simulink model "dSAW"  (R2019a)
settings: Solver=FixedStepAuto  StartTime=0.0  StopTime=40  FixedStep=0.001  MaxStep=0.01  RelTol=1e-3  AbsTol=1e-3  EnableMultiTasking=on
values from neighbouring files (symbols this model uses):
  alp = data(:,1)    [Main.m]
  be_gap = 23    [Main.m]
  cd = data(:,3)    [Main.m]
  chord_lengths = [61.1183,64.3430,68.0127,71.9324,                 75.9071,79.7418,83.2415,86.2112,                 88.4559,89.7806,89.9903,88.8900]    [Main.m]
  cl = data(:,2)    [Main.m]
  epsilon = 0.2010    (= 0.201)    [Main.m]
  gamma_amp = 0.1188    [Main.m]
  gamma_o = -0.1345    [Main.m]
undefined symbols (not defined in the file or in its folder): X, Y, Z
libraries: sm_lib x168, nesl_utility x109, dspindex x2
(part 3 of 3)

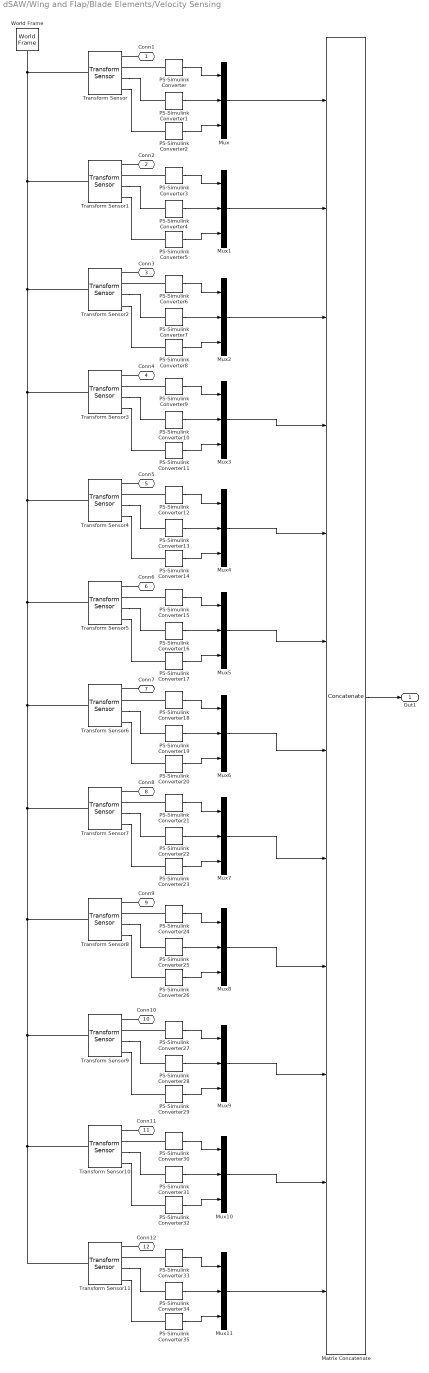
== system dSAW/Wing and Flap/Blade Elements/Velocity Sensing ==
  Matrix Concatenate : Concatenate  NumInputs=12  Mode=Multidimensional array  ConcatenateDimension=2
  Mux{,1..11} (12 alike) : Mux  Inputs=3
  PS-Simulink Converter{,1..35} (36 alike) : nesl_utility/PS-Simulink Converter  PhysicalDomain=network_engine_domain  SubClassName=ps_output  LeftPortType=input  RightPortType=output  PseudoPeriodic=off  Frequencies=[]  Unit=1  AffineConversion=off
  Transform Sensor{,1..11} (12 alike) : sm_lib/Frames and Transforms/Transform Sensor  MeasurementFrame=NonRotatingFollower  SenseAngle=off  SenseAxis=off  SenseAngle1=off  SenseAngle2=off  SenseAngle3=off  SenseQ=off  SenseR=off  SenseOmegaX=off  SenseOmegaY=off  SenseOmegaZ=off  SenseOmega1=off  SenseOmega2=off  SenseOmega3=off  SenseQDot=off  SenseRDot=off  SenseAlphaX=off  SenseAlphaY=off  SenseAlphaZ=off  SenseAlpha1=off  SenseAlpha2=off  SenseAlpha3=off  SenseQDDot=off  SenseRDDot=off  SenseX=off  SenseY=off  SenseZ=off  SenseRad=off  SenseAzim=off  SenseDist=off  SenseInc=off  SenseXDot=on  SenseYDot=on  SenseZDot=on  SenseRadDot=off  SenseAzimDot=off  SenseDistDot=off  SenseIncDot=off  SenseXDDot=off  SenseYDDot=off  SenseZDDot=off  SenseRadDDot=off  SenseAzimDDot=off  SenseDistDDot=off  SenseIncDDot=off
  World Frame : sm_lib/Frames and Transforms/World Frame
  Conn1 : PMIOPort  Side=Left
  Conn2 : PMIOPort  Port=2  Side=Left
  Conn3 : PMIOPort  Port=3  Side=Left
  Conn4 : PMIOPort  Port=4  Side=Left
  Conn5 : PMIOPort  Port=5  Side=Left
  Conn6 : PMIOPort  Port=6  Side=Left
  Conn7 : PMIOPort  Port=7  Side=Left
  Conn8 : PMIOPort  Port=8  Side=Left
  Conn9 : PMIOPort  Port=9  Side=Left
  Conn10 : PMIOPort  Port=10  Side=Left
  Conn11 : PMIOPort  Port=11  Side=Left
  Conn12 : PMIOPort  Port=12  Side=Left
  Out1 : Outport
  wires:
  PS-Simulink Converter1/1 -> Mux/2
  PS-Simulink Converter/1 -> Mux/1
  PS-Simulink Converter2/1 -> Mux/3
  Matrix Concatenate/1 -> Out1/1
  Mux/1 -> Matrix Concatenate/1
  Mux1/1 -> Matrix Concatenate/2
  PS-Simulink Converter3/1 -> Mux1/1
  PS-Simulink Converter4/1 -> Mux1/2
  PS-Simulink Converter5/1 -> Mux1/3
  PS-Simulink Converter6/1 -> Mux2/1
  PS-Simulink Converter7/1 -> Mux2/2
  PS-Simulink Converter8/1 -> Mux2/3
  PS-Simulink Converter9/1 -> Mux3/1
  PS-Simulink Converter10/1 -> Mux3/2
  PS-Simulink Converter11/1 -> Mux3/3
  PS-Simulink Converter12/1 -> Mux4/1
  PS-Simulink Converter13/1 -> Mux4/2
  PS-Simulink Converter14/1 -> Mux4/3
  PS-Simulink Converter15/1 -> Mux5/1
  PS-Simulink Converter16/1 -> Mux5/2
  PS-Simulink Converter17/1 -> Mux5/3
  PS-Simulink Converter18/1 -> Mux6/1
  PS-Simulink Converter19/1 -> Mux6/2
  PS-Simulink Converter20/1 -> Mux6/3
  PS-Simulink Converter21/1 -> Mux7/1
  PS-Simulink Converter22/1 -> Mux7/2
  PS-Simulink Converter23/1 -> Mux7/3
  Mux2/1 -> Matrix Concatenate/3
  Mux3/1 -> Matrix Concatenate/4
  Mux4/1 -> Matrix Concatenate/5
  Mux5/1 -> Matrix Concatenate/6
  Mux6/1 -> Matrix Concatenate/7
  Mux7/1 -> Matrix Concatenate/8
  PS-Simulink Converter26/1 -> Mux8/3
  PS-Simulink Converter25/1 -> Mux8/2
  PS-Simulink Converter24/1 -> Mux8/1
  PS-Simulink Converter27/1 -> Mux9/1
  PS-Simulink Converter28/1 -> Mux9/2
  PS-Simulink Converter29/1 -> Mux9/3
  PS-Simulink Converter32/1 -> Mux10/3
  PS-Simulink Converter31/1 -> Mux10/2
  PS-Simulink Converter30/1 -> Mux10/1
  Mux8/1 -> Matrix Concatenate/9
  Mux9/1 -> Matrix Concatenate/10
  Mux10/1 -> Matrix Concatenate/11
  Mux11/1 -> Matrix Concatenate/12
  PS-Simulink Converter33/1 -> Mux11/1
  PS-Simulink Converter34/1 -> Mux11/2
  PS-Simulink Converter35/1 -> Mux11/3
  connections:
  Transform Sensor/LConn1 -- Transform Sensor11/LConn1 -- Transform Sensor10/LConn1 -- Transform Sensor9/LConn1 -- Transform Sensor8/LConn1 -- Transform Sensor7/LConn1 -- Transform Sensor6/LConn1 -- Transform Sensor5/LConn1 -- Transform Sensor4/LConn1 -- Transform Sensor3/LConn1 -- Transform Sensor2/LConn1 -- Transform Sensor1/LConn1 -- World Frame/RConn1
  Conn1/RConn1 -- Transform Sensor/RConn1
  PS-Simulink Converter/LConn1 -- Transform Sensor/RConn2
  Transform Sensor/RConn3 -- PS-Simulink Converter1/LConn1
  Transform Sensor/RConn4 -- PS-Simulink Converter2/LConn1
  Transform Sensor1/RConn4 -- PS-Simulink Converter5/LConn1
  PS-Simulink Converter3/LConn1 -- Transform Sensor1/RConn2
  Transform Sensor1/RConn3 -- PS-Simulink Converter4/LConn1
  Conn2/RConn1 -- Transform Sensor1/RConn1
  PS-Simulink Converter6/LConn1 -- Transform Sensor2/RConn2
  Transform Sensor2/RConn4 -- PS-Simulink Converter8/LConn1
  Transform Sensor2/RConn3 -- PS-Simulink Converter7/LConn1
  PS-Simulink Converter9/LConn1 -- Transform Sensor3/RConn2
  Transform Sensor3/RConn4 -- PS-Simulink Converter11/LConn1
  Transform Sensor3/RConn3 -- PS-Simulink Converter10/LConn1
  PS-Simulink Converter12/LConn1 -- Transform Sensor4/RConn2
  Transform Sensor4/RConn4 -- PS-Simulink Converter14/LConn1
  Transform Sensor4/RConn3 -- PS-Simulink Converter13/LConn1
  PS-Simulink Converter15/LConn1 -- Transform Sensor5/RConn2
  Transform Sensor5/RConn4 -- PS-Simulink Converter17/LConn1
  Transform Sensor5/RConn3 -- PS-Simulink Converter16/LConn1
  PS-Simulink Converter18/LConn1 -- Transform Sensor6/RConn2
  Transform Sensor6/RConn4 -- PS-Simulink Converter20/LConn1
  Transform Sensor6/RConn3 -- PS-Simulink Converter19/LConn1
  PS-Simulink Converter21/LConn1 -- Transform Sensor7/RConn2
  Transform Sensor7/RConn4 -- PS-Simulink Converter23/LConn1
  Transform Sensor7/RConn3 -- PS-Simulink Converter22/LConn1
  Conn3/RConn1 -- Transform Sensor2/RConn1
  Conn4/RConn1 -- Transform Sensor3/RConn1
  Conn5/RConn1 -- Transform Sensor4/RConn1
  Conn6/RConn1 -- Transform Sensor5/RConn1
  Conn7/RConn1 -- Transform Sensor6/RConn1
  Conn8/RConn1 -- Transform Sensor7/RConn1
  Conn9/RConn1 -- Transform Sensor8/RConn1
  Transform Sensor8/RConn3 -- PS-Simulink Converter25/LConn1
  Transform Sensor8/RConn4 -- PS-Simulink Converter26/LConn1
  PS-Simulink Converter24/LConn1 -- Transform Sensor8/RConn2
  PS-Simulink Converter27/LConn1 -- Transform Sensor9/RConn2
  Transform Sensor9/RConn4 -- PS-Simulink Converter29/LConn1
  Transform Sensor9/RConn3 -- PS-Simulink Converter28/LConn1
  Conn10/RConn1 -- Transform Sensor9/RConn1
  Transform Sensor10/RConn3 -- PS-Simulink Converter31/LConn1
  Transform Sensor10/RConn4 -- PS-Simulink Converter32/LConn1
  Conn11/RConn1 -- Transform Sensor10/RConn1
  PS-Simulink Converter30/LConn1 -- Transform Sensor10/RConn2
  Conn12/RConn1 -- Transform Sensor11/RConn1
  PS-Simulink Converter33/LConn1 -- Transform Sensor11/RConn2
  Transform Sensor11/RConn4 -- PS-Simulink Converter35/LConn1
  Transform Sensor11/RConn3 -- PS-Simulink Converter34/LConn1

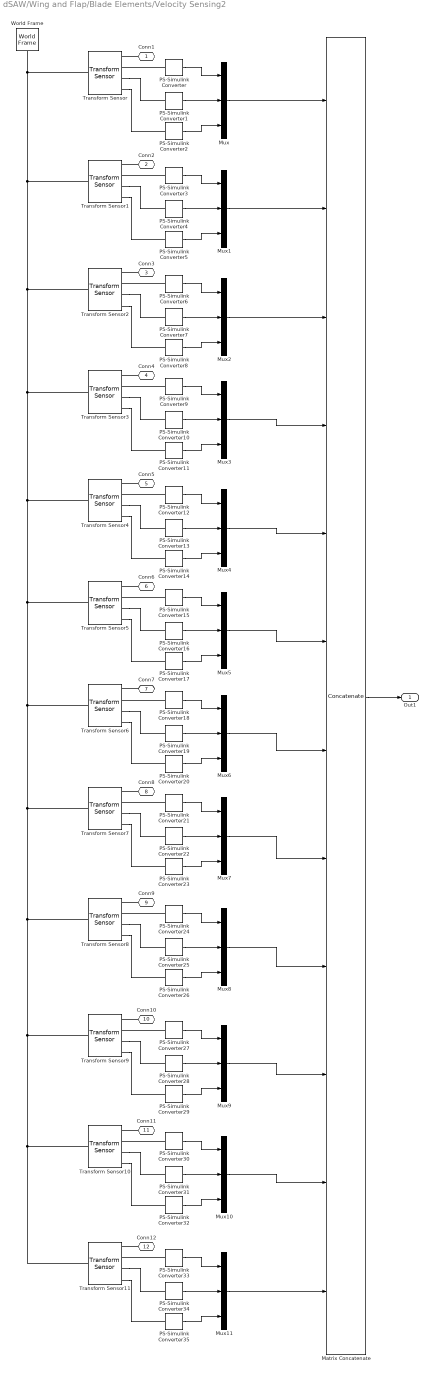
== system dSAW/Wing and Flap/Blade Elements/Velocity Sensing2 ==
  Matrix Concatenate : Concatenate  NumInputs=12  Mode=Multidimensional array  ConcatenateDimension=2
  Mux{,1..11} (12 alike) : Mux  Inputs=3
  PS-Simulink Converter{,1..35} (36 alike) : nesl_utility/PS-Simulink Converter  PhysicalDomain=network_engine_domain  SubClassName=ps_output  LeftPortType=input  RightPortType=output  PseudoPeriodic=off  Frequencies=[]  Unit=1  AffineConversion=off
  Transform Sensor{,1..11} (12 alike) : sm_lib/Frames and Transforms/Transform Sensor  MeasurementFrame=NonRotatingFollower  SenseAngle=off  SenseAxis=off  SenseAngle1=off  SenseAngle2=off  SenseAngle3=off  SenseQ=off  SenseR=off  SenseOmegaX=off  SenseOmegaY=off  SenseOmegaZ=off  SenseOmega1=off  SenseOmega2=off  SenseOmega3=off  SenseQDot=off  SenseRDot=off  SenseAlphaX=off  SenseAlphaY=off  SenseAlphaZ=off  SenseAlpha1=off  SenseAlpha2=off  SenseAlpha3=off  SenseQDDot=off  SenseRDDot=off  SenseX=off  SenseY=off  SenseZ=off  SenseRad=off  SenseAzim=off  SenseDist=off  SenseInc=off  SenseXDot=on  SenseYDot=on  SenseZDot=on  SenseRadDot=off  SenseAzimDot=off  SenseDistDot=off  SenseIncDot=off  SenseXDDot=off  SenseYDDot=off  SenseZDDot=off  SenseRadDDot=off  SenseAzimDDot=off  SenseDistDDot=off  SenseIncDDot=off
  World Frame : sm_lib/Frames and Transforms/World Frame
  Conn1 : PMIOPort  Side=Left
  Conn2 : PMIOPort  Port=2  Side=Left
  Conn3 : PMIOPort  Port=3  Side=Left
  Conn4 : PMIOPort  Port=4  Side=Left
  Conn5 : PMIOPort  Port=5  Side=Left
  Conn6 : PMIOPort  Port=6  Side=Left
  Conn7 : PMIOPort  Port=7  Side=Left
  Conn8 : PMIOPort  Port=8  Side=Left
  Conn9 : PMIOPort  Port=9  Side=Left
  Conn10 : PMIOPort  Port=10  Side=Left
  Conn11 : PMIOPort  Port=11  Side=Left
  Conn12 : PMIOPort  Port=12  Side=Left
  Out1 : Outport
  wires:
  PS-Simulink Converter1/1 -> Mux/2
  PS-Simulink Converter/1 -> Mux/1
  PS-Simulink Converter2/1 -> Mux/3
  Matrix Concatenate/1 -> Out1/1
  Mux/1 -> Matrix Concatenate/1
  Mux1/1 -> Matrix Concatenate/2
  PS-Simulink Converter3/1 -> Mux1/1
  PS-Simulink Converter4/1 -> Mux1/2
  PS-Simulink Converter5/1 -> Mux1/3
  PS-Simulink Converter6/1 -> Mux2/1
  PS-Simulink Converter7/1 -> Mux2/2
  PS-Simulink Converter8/1 -> Mux2/3
  PS-Simulink Converter9/1 -> Mux3/1
  PS-Simulink Converter10/1 -> Mux3/2
  PS-Simulink Converter11/1 -> Mux3/3
  PS-Simulink Converter12/1 -> Mux4/1
  PS-Simulink Converter13/1 -> Mux4/2
  PS-Simulink Converter14/1 -> Mux4/3
  PS-Simulink Converter15/1 -> Mux5/1
  PS-Simulink Converter16/1 -> Mux5/2
  PS-Simulink Converter17/1 -> Mux5/3
  PS-Simulink Converter18/1 -> Mux6/1
  PS-Simulink Converter19/1 -> Mux6/2
  PS-Simulink Converter20/1 -> Mux6/3
  PS-Simulink Converter21/1 -> Mux7/1
  PS-Simulink Converter22/1 -> Mux7/2
  PS-Simulink Converter23/1 -> Mux7/3
  Mux2/1 -> Matrix Concatenate/3
  Mux3/1 -> Matrix Concatenate/4
  Mux4/1 -> Matrix Concatenate/5
  Mux5/1 -> Matrix Concatenate/6
  Mux6/1 -> Matrix Concatenate/7
  Mux7/1 -> Matrix Concatenate/8
  PS-Simulink Converter26/1 -> Mux8/3
  PS-Simulink Converter25/1 -> Mux8/2
  PS-Simulink Converter24/1 -> Mux8/1
  PS-Simulink Converter27/1 -> Mux9/1
  PS-Simulink Converter28/1 -> Mux9/2
  PS-Simulink Converter29/1 -> Mux9/3
  PS-Simulink Converter32/1 -> Mux10/3
  PS-Simulink Converter31/1 -> Mux10/2
  PS-Simulink Converter30/1 -> Mux10/1
  Mux8/1 -> Matrix Concatenate/9
  Mux9/1 -> Matrix Concatenate/10
  Mux10/1 -> Matrix Concatenate/11
  Mux11/1 -> Matrix Concatenate/12
  PS-Simulink Converter33/1 -> Mux11/1
  PS-Simulink Converter34/1 -> Mux11/2
  PS-Simulink Converter35/1 -> Mux11/3
  connections:
  Transform Sensor/LConn1 -- Transform Sensor11/LConn1 -- Transform Sensor10/LConn1 -- Transform Sensor9/LConn1 -- Transform Sensor8/LConn1 -- Transform Sensor7/LConn1 -- Transform Sensor6/LConn1 -- Transform Sensor5/LConn1 -- Transform Sensor4/LConn1 -- Transform Sensor3/LConn1 -- Transform Sensor2/LConn1 -- Transform Sensor1/LConn1 -- World Frame/RConn1
  Conn1/RConn1 -- Transform Sensor/RConn1
  PS-Simulink Converter/LConn1 -- Transform Sensor/RConn2
  Transform Sensor/RConn3 -- PS-Simulink Converter1/LConn1
  Transform Sensor/RConn4 -- PS-Simulink Converter2/LConn1
  Transform Sensor1/RConn4 -- PS-Simulink Converter5/LConn1
  PS-Simulink Converter3/LConn1 -- Transform Sensor1/RConn2
  Transform Sensor1/RConn3 -- PS-Simulink Converter4/LConn1
  Conn2/RConn1 -- Transform Sensor1/RConn1
  PS-Simulink Converter6/LConn1 -- Transform Sensor2/RConn2
  Transform Sensor2/RConn4 -- PS-Simulink Converter8/LConn1
  Transform Sensor2/RConn3 -- PS-Simulink Converter7/LConn1
  PS-Simulink Converter9/LConn1 -- Transform Sensor3/RConn2
  Transform Sensor3/RConn4 -- PS-Simulink Converter11/LConn1
  Transform Sensor3/RConn3 -- PS-Simulink Converter10/LConn1
  PS-Simulink Converter12/LConn1 -- Transform Sensor4/RConn2
  Transform Sensor4/RConn4 -- PS-Simulink Converter14/LConn1
  Transform Sensor4/RConn3 -- PS-Simulink Converter13/LConn1
  PS-Simulink Converter15/LConn1 -- Transform Sensor5/RConn2
  Transform Sensor5/RConn4 -- PS-Simulink Converter17/LConn1
  Transform Sensor5/RConn3 -- PS-Simulink Converter16/LConn1
  PS-Simulink Converter18/LConn1 -- Transform Sensor6/RConn2
  Transform Sensor6/RConn4 -- PS-Simulink Converter20/LConn1
  Transform Sensor6/RConn3 -- PS-Simulink Converter19/LConn1
  PS-Simulink Converter21/LConn1 -- Transform Sensor7/RConn2
  Transform Sensor7/RConn4 -- PS-Simulink Converter23/LConn1
  Transform Sensor7/RConn3 -- PS-Simulink Converter22/LConn1
  Conn3/RConn1 -- Transform Sensor2/RConn1
  Conn4/RConn1 -- Transform Sensor3/RConn1
  Conn5/RConn1 -- Transform Sensor4/RConn1
  Conn6/RConn1 -- Transform Sensor5/RConn1
  Conn7/RConn1 -- Transform Sensor6/RConn1
  Conn8/RConn1 -- Transform Sensor7/RConn1
  Conn9/RConn1 -- Transform Sensor8/RConn1
  Transform Sensor8/RConn3 -- PS-Simulink Converter25/LConn1
  Transform Sensor8/RConn4 -- PS-Simulink Converter26/LConn1
  PS-Simulink Converter24/LConn1 -- Transform Sensor8/RConn2
  PS-Simulink Converter27/LConn1 -- Transform Sensor9/RConn2
  Transform Sensor9/RConn4 -- PS-Simulink Converter29/LConn1
  Transform Sensor9/RConn3 -- PS-Simulink Converter28/LConn1
  Conn10/RConn1 -- Transform Sensor9/RConn1
  Transform Sensor10/RConn3 -- PS-Simulink Converter31/LConn1
  Transform Sensor10/RConn4 -- PS-Simulink Converter32/LConn1
  Conn11/RConn1 -- Transform Sensor10/RConn1
  PS-Simulink Converter30/LConn1 -- Transform Sensor10/RConn2
  Conn12/RConn1 -- Transform Sensor11/RConn1
  PS-Simulink Converter33/LConn1 -- Transform Sensor11/RConn2
  Transform Sensor11/RConn4 -- PS-Simulink Converter35/LConn1
  Transform Sensor11/RConn3 -- PS-Simulink Converter34/LConn1

== matlab function dSAW/Wing and Flap/BET ==
  data: U input; fx output; CL input; CD input; alpha input; fz output; F output; be_gap input; dL output; dD output
function [fx, fz, F, dL, dD] = bet(U, CL, CD, alpha, be_gap)

dL = zeros(12,1);
dD = zeros(12,1);
fx = zeros(12,1);
fy = zeros(12,1);
fz = zeros(12,1);

rho = 1.225;        % density of air
dy = 0.001 * be_gap;  

for i = 1:12
    dL(i) = 0.5 * rho * U(i)^2 * 0.001 * 38 * CL(i) * dy;
    dD(i) = 0.5 * rho * U(i)^2 * 0.001 * 38 * CD(i) * dy;
    fx(i) = dL(i) * sin(alpha(i)) - dD(i) * cos(alpha(i));
    fz(i) = dL(i) * cos(alpha(i)) + dD(i) * sin(alpha(i));
end

F = [-fx fy fz];

== matlab function dSAW/Wing and Flap/Read Velocity ==
  data: aerovels input; vx output; vy output; vz output; U output; alpha output
function [vx, vy, vz, U, alpha] = readvel(aerovels)

vx = aerovels(1,:);
vy = aerovels(2,:);
vz = aerovels(3,:);

U = sqrt(vx.^2 + vz.^2);
alpha = atan(-vz./abs(vx));

== matlab function dSAW/Wing and Flap/BET1 ==
  data: U input; fx output; CL input; CD input; alpha input; fz output; F output; chord input; be_gap input
function [fx, fz, F] = bet(U, CL, CD, alpha, chord, be_gap)

dL = zeros(11,1);
dD = zeros(11,1);
fx = zeros(11,1);
fy = zeros(11,1);
fz = zeros(11,1);

rho = 1.225;        % density of air
dy =  0.001 * be_gap;   

for i = 1:11
    dL(i) = 0.5 * rho * U(i)^2 * 0.001 * chord(i) * CL(i) * dy;
    dD(i) = 0.5 * rho * U(i)^2 * 0.001 * chord(i) * CD(i) * dy;
    fx(i) = dL(i) * sin(alpha(i)) - dD(i) * cos(alpha(i));
    fz(i) = dL(i) * cos(alpha(i)) + dD(i) * sin(alpha(i));
end

F = [-fx fy fz];

== matlab function dSAW/Wing and Flap/Read Velocity1 ==
  data: aerovels input; vx output; vy output; vz output; U output; alpha output
function [vx, vy, vz, U, alpha] = readvel(aerovels)

vx = aerovels(1,:);
vy = aerovels(2,:);
vz = aerovels(3,:);

U = sqrt(vx.^2 + vz.^2);
alpha = atan(-vz./abs(vx));

== matlab function dSAW/Direction Finder ==
  data: t input; dir output; pitch input; roll input; mag output
function [dir, mag] = direction(t, pitch, roll)

dir = atan2(pitch, roll);
mag = sqrt(roll^2 + pitch^2);

if mag > 1
    mag = 1;
end

== matlab function dSAW/Swash ==
  settings: updateMethod=DISCRETE
  data: t input; quat input; flap output; quatold input; dir input; mag input; azimuth output; gamma_o input; epsilon input; gamma_amp input
function [flap, azimuth] = swash(t, quat, quatold, dir, mag, gamma_o, epsilon, gamma_amp)

if quat < quatold
        y = sin(quat);
        x = -cos(quat);
        azimuth = atan2(y,x) + pi;
else
        azimuth = quat;
end

flap = -0.1887;
offset = -2.2;

azimuth = azimuth * 2;
if azimuth > 2*pi
    azimuth = azimuth - 2*pi;
end

if t > 10
    flap =  gamma_o;
    if sin(azimuth + dir + offset) > epsilon
        flap = flap + mag * gamma_amp;
    elseif sin(azimuth + dir + offset) < -epsilon
        flap = flap - mag * gamma_amp;
    end
%     flap = gamma_o + mag * gamma_amp * sin(azimuth + dir + offset); %%
%     uncomment for sinusoidal cyclic control
end

== matlab function dSAW/MATLAB Function ==
  data: x input; r output; y input
function r = dist(x, y)

r = sqrt(x^2 + y^2);
